simulink model "SC_Eco_5_5"  (R2013a)
settings: Solver=FixedStepDiscrete  StartTime=0.0  StopTime=800  RelTol=1e-3
values from neighbouring files (symbols this model uses):
  T = 1    [Variaveis.mat]
undefined symbols (not defined in the file or in its folder): mu, St
settings Model: Creator=Élio  LastModifiedBy=Élio

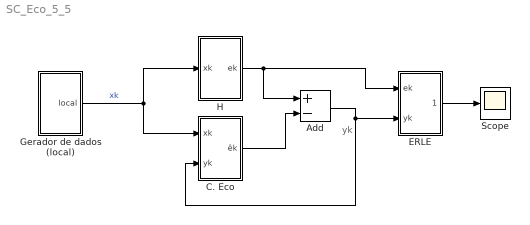
== system SC_Eco_5_5 ==
  note: yk
  Add : Sum  Inputs=+-
  C. Eco : Subsystem
  ERLE : Subsystem
  Gerador de dados (local) : Subsystem
  H : Subsystem
  "Scope " : Scope
  wires:
  Gerador de dados (local)/1(local) -> C. Eco/1(xk), H/1(xk)  "xk"
  C. Eco/1(êk) -> Add/2
  ERLE/1(ERLE) -> "Scope "/1
  H/1(ek) -> ERLE/1(ek), Add/1
  Add/1 -> ERLE/2(yk), C. Eco/2(yk)

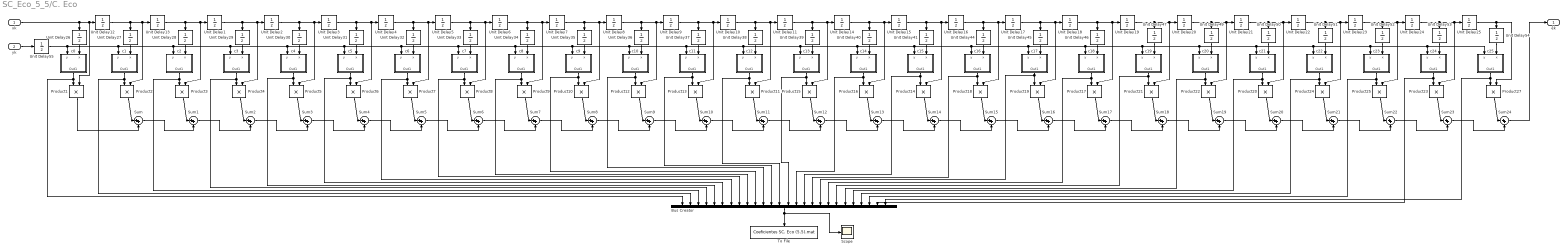
== system SC_Eco_5_5/C. Eco ==
  xk : Inport
  yk : Inport  Port=2
  Bus Creator : BusCreator  Inputs=26
  Product{1..25,27} (26 alike) : Product
  Scope : Scope
  Sum{,1..24} (25 alike) : Sum  Inputs=|++
  To File : ToFile  Filename=Coeficientes SC. Eco (5.5).mat  MatrixName=c5_5  SaveFormat=Timeseries
  Unit Delay{1..41,44..47,49..55} (52 alike) : UnitDelay  SampleTime=-1
  c0 : Subsystem
  c1 : Subsystem
  c10 : Subsystem
  c11 : Subsystem
  c12 : Subsystem
  c13 : Subsystem
  c14 : Subsystem
  c15 : Subsystem
  c16 : Subsystem
  c17 : Subsystem
  c18 : Subsystem
  c19 : Subsystem
  c2 : Subsystem
  c20 : Subsystem
  c21 : Subsystem
  c22 : Subsystem
  c23 : Subsystem
  c24 : Subsystem
  c25 : Subsystem
  c3 : Subsystem
  c4 : Subsystem
  c5 : Subsystem
  c6 : Subsystem
  c7 : Subsystem
  c8 : Subsystem
  c9 : Subsystem
  êk : Outport
  wires:
  Sum/1 -> Sum1/2
  Product1/1 -> Sum/2
  Product2/1 -> Sum/1
  Unit Delay12/1 -> Unit Delay27/1, Product2/2, Unit Delay13/1
  Product3/1 -> Sum1/1
  Product4/1 -> Sum2/1
  Unit Delay13/1 -> Unit Delay1/1, Product3/2, Unit Delay28/1
  Sum2/1 -> Sum3/2
  Product6/1 -> Sum4/1
  xk/1 -> Product1/2, Unit Delay12/1, Unit Delay26/1
  Product5/1 -> Sum3/1
  Sum3/1 -> Sum4/2
  Sum4/1 -> Sum5/2
  Product7/1 -> Sum5/1
  Unit Delay4/1 -> Unit Delay5/1, Product7/2, Unit Delay32/1
  Unit Delay2/1 -> Unit Delay3/1, Product5/2, Unit Delay30/1
  Unit Delay3/1 -> Unit Delay4/1, Product6/2, Unit Delay31/1
  Sum5/1 -> Sum6/2
  Unit Delay5/1 -> Unit Delay6/1, Product8/2, Unit Delay33/1
  Product9/1 -> Sum7/1
  Unit Delay6/1 -> Unit Delay7/1, Product9/2, Unit Delay34/1
  Sum1/1 -> Sum2/2
  Product8/1 -> Sum6/1
  Sum7/1 -> Sum8/2
  Product10/1 -> Sum8/1
  Unit Delay1/1 -> Unit Delay2/1, Product4/2, Unit Delay29/1
  Sum6/1 -> Sum7/2
  Product12/1 -> Sum9/1
  Unit Delay11/1 -> Unit Delay14/1, Product15/2, Unit Delay39/1
  Unit Delay10/1 -> Unit Delay11/1, Product11/2, Unit Delay38/1
  Unit Delay9/1 -> Unit Delay10/1, Product13/2, Unit Delay37/1
  Product11/1 -> Sum11/1
  Product13/1 -> Sum10/1
  Sum12/1 -> Sum13/2
  Product15/1 -> Sum12/1
  Sum9/1 -> Sum10/2
  Product16/1 -> Sum13/1
  Sum11/1 -> Sum12/2
  Sum8/1 -> Sum9/2
  Unit Delay8/1 -> Unit Delay9/1, Product12/2, Unit Delay36/1
  Sum10/1 -> Sum11/2
  Sum13/1 -> Sum14/2
  Unit Delay7/1 -> Unit Delay8/1, Product10/2, Unit Delay35/1
  Unit Delay14/1 -> Unit Delay15/1, Product16/2, Unit Delay40/1
  Product14/1 -> Sum14/1
  Unit Delay17/1 -> Unit Delay18/1, Product19/2, Unit Delay45/1
  Product18/1 -> Sum15/1
  Unit Delay19/1 -> Unit Delay20/1, Product21/2, Unit Delay47/1
  Unit Delay15/1 -> Unit Delay16/1, Product14/2, Unit Delay41/1
  Sum18/1 -> Sum19/2
  Sum16/1 -> Sum17/2
  Product19/1 -> Sum16/1
  Sum21/1 -> Sum22/2
  Sum15/1 -> Sum16/2
  Unit Delay16/1 -> Unit Delay17/1, Product18/2, Unit Delay44/1
  Unit Delay20/1 -> Unit Delay21/1, Product22/2, Unit Delay49/1
  Product21/1 -> Sum18/1
  Sum17/1 -> Sum18/2
  Sum14/1 -> Sum15/2
  Sum19/1 -> Sum20/2
  Product17/1 -> Sum17/1
  Unit Delay22/1 -> Unit Delay23/1, Product24/2, Unit Delay51/1
  Product20/1 -> Sum20/1
  Product24/1 -> Sum21/1
  Unit Delay21/1 -> Unit Delay22/1, Product20/2, Unit Delay50/1
  Sum20/1 -> Sum21/2
  Unit Delay18/1 -> Unit Delay19/1, Product17/2, Unit Delay46/1
  Product22/1 -> Sum19/1
  Unit Delay40/1 -> c14/2(x)
  Unit Delay32/1 -> c6/2(x)
  Product23/1 -> Sum23/1
  Unit Delay24/1 -> Unit Delay25/1, Product23/2, Unit Delay53/1
  Product25/1 -> Sum22/1
  Unit Delay27/1 -> c1/2(x)
  Unit Delay26/1 -> c0/2(x)
  Unit Delay33/1 -> c7/2(x)
  Unit Delay34/1 -> c8/2(x)
  Unit Delay23/1 -> Unit Delay24/1, Product25/2, Unit Delay52/1
  Sum23/1 -> Sum24/2
  Unit Delay28/1 -> c2/2(x)
  Unit Delay35/1 -> c9/2(x)
  Unit Delay36/1 -> c10/2(x)
  Unit Delay44/1 -> c16/2(x)
  Unit Delay45/1 -> c17/2(x)
  Unit Delay46/1 -> c18/2(x)
  Unit Delay25/1 -> Product27/2, Unit Delay54/1
  yk/1 -> Unit Delay55/1
  Sum24/1 -> êk/1
  Unit Delay31/1 -> c5/2(x)
  Unit Delay39/1 -> c13/2(x)
  Unit Delay30/1 -> c4/2(x)
  Unit Delay38/1 -> c12/2(x)
  Unit Delay41/1 -> c15/2(x)
  Unit Delay29/1 -> c3/2(x)
  Unit Delay37/1 -> c11/2(x)
  Sum22/1 -> Sum23/2
  Product27/1 -> Sum24/1
  Unit Delay53/1 -> c24/2(x)
  Unit Delay47/1 -> c19/2(x)
  Unit Delay54/1 -> c25/2(x)
  Unit Delay49/1 -> c20/2(x)
  Unit Delay50/1 -> c21/2(x)
  Unit Delay55/1 -> c0/1(y), c1/1(y), c2/1(y), c3/1(y), c4/1(y), c5/1(y), c6/1(y), c7/1(y), c8/1(y), c9/1(y), c10/1(y), c11/1(y), c12/1(y), c14/1(y), c15/1(y), c16/1(y), c17/1(y), c18/1(y), c19/1(y), c20/1(y), c21/1(y), c22/1(y), c23/1(y), c25/1(y), c24/1(y), c13/1(y)
  Unit Delay52/1 -> c23/2(x)
  Unit Delay51/1 -> c22/2(x)
  c1/1(Out1) -> Bus Creator/2, Product2/1
  c0/1(Out1) -> Bus Creator/1, Product1/1
  c2/1(Out1) -> Bus Creator/3, Product3/1
  c3/1(Out1) -> Bus Creator/4, Product4/1
  c4/1(Out1) -> Bus Creator/5, Product5/1
  c5/1(Out1) -> Bus Creator/6, Product6/1
  c6/1(Out1) -> Bus Creator/7, Product7/1
  c7/1(Out1) -> Bus Creator/8, Product8/1
  c8/1(Out1) -> Bus Creator/9, Product9/1
  c9/1(Out1) -> Bus Creator/10, Product10/1
  c10/1(Out1) -> Bus Creator/11, Product12/1
  c11/1(Out1) -> Bus Creator/12, Product13/1
  c12/1(Out1) -> Bus Creator/13, Product11/1
  c13/1(Out1) -> Bus Creator/14, Product15/1
  c14/1(Out1) -> Bus Creator/15, Product16/1
  c15/1(Out1) -> Bus Creator/16, Product14/1
  c16/1(Out1) -> Bus Creator/17, Product18/1
  c17/1(Out1) -> Bus Creator/18, Product19/1
  c18/1(Out1) -> Bus Creator/19, Product17/1
  c19/1(Out1) -> Bus Creator/20, Product21/1
  c20/1(Out1) -> Bus Creator/21, Product22/1
  c21/1(Out1) -> Bus Creator/22, Product20/1
  c22/1(Out1) -> Bus Creator/23, Product24/1
  c23/1(Out1) -> Bus Creator/24, Product25/1
  c24/1(Out1) -> Bus Creator/25, Product23/1
  c25/1(Out1) -> Bus Creator/26, Product27/1
  Bus Creator/1 -> Scope/1, To File/1

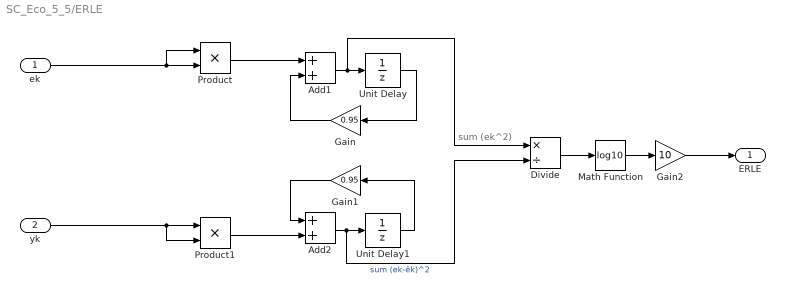
== system SC_Eco_5_5/ERLE ==
  note: sum (ek^2)
  ek : Inport
  yk : Inport  Port=2
  Add1 : Sum  RequirementInfo={} %GIDa_ce1c1d54_3b96_46b2_aaba_1a46e1338465
  Add2 : Sum  RequirementInfo={} %GIDa_00d8fe9e_6752_48b6_b576_e88cd44475ea
  Divide : Product  Inputs=*/
  Gain : Gain  Gain=0.95
  Gain1 : Gain  Gain=0.95
  Gain2 : Gain  Gain=10
  Math Function : Math  Operator=log10  SaturateOnIntegerOverflow=on
  Product : Product
  Product1 : Product
  Unit Delay : UnitDelay  SampleTime=-1
  Unit Delay1 : UnitDelay  SampleTime=-1
  ERLE : Outport
  wires:
  yk/1 -> Product1/2, Product1/1
  Math Function/1 -> Gain2/1
  Add2/1 -> Divide/2, Unit Delay1/1  "sum (ek-êk)^2"
  Product/1 -> Add1/1
  Gain1/1 -> Add2/1
  Divide/1 -> Math Function/1
  Gain2/1 -> ERLE/1
  Unit Delay1/1 -> Gain1/1
  Add1/1 -> Divide/1, Unit Delay/1
  Unit Delay/1 -> Gain/1
  ek/1 -> Product/2, Product/1
  Gain/1 -> Add1/2
  Product1/1 -> Add2/2

== system SC_Eco_5_5/Gerador de dados (local) ==
  Conversor de nível : Subsystem
  Pulse Generator : DiscretePulseGenerator  PulseType=Time based  Period=2*T  PulseWidth=50  SampleTime=St
  Scrambler (local) : Subsystem
  local : Outport
  wires:
  Pulse Generator/1 -> Scrambler (local)/1(In1)
  Conversor de nível/1(Out2) -> local/1
  Scrambler (local)/1(Out1) -> Conversor de nível/1(In2)

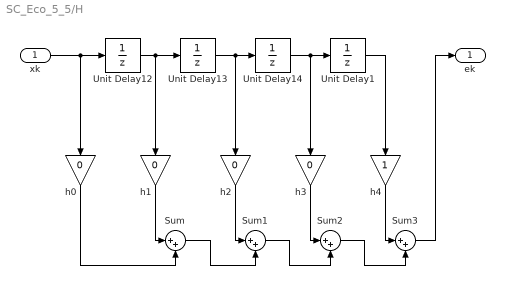
== system SC_Eco_5_5/H ==
  xk : Inport
  Sum{,1..3} (4 alike) : Sum  Inputs=|++
  Unit Delay{1,12..14} (4 alike) : UnitDelay  SampleTime=-1
  h{0..3} (4 alike) : Gain  Gain=0
  h4 : Gain
  ek : Outport
  wires:
  Sum3/1 -> ek/1
  xk/1 -> Unit Delay12/1, h0/1
  Unit Delay13/1 -> Unit Delay14/1, h2/1
  h3/1 -> Sum2/1
  Unit Delay14/1 -> Unit Delay1/1, h3/1
  Sum/1 -> Sum1/2
  h2/1 -> Sum1/1
  h0/1 -> Sum/2
  Unit Delay12/1 -> Unit Delay13/1, h1/1
  Sum1/1 -> Sum2/2
  h1/1 -> Sum/1
  Unit Delay1/1 -> h4/1
  Sum2/1 -> Sum3/2
  h4/1 -> Sum3/1

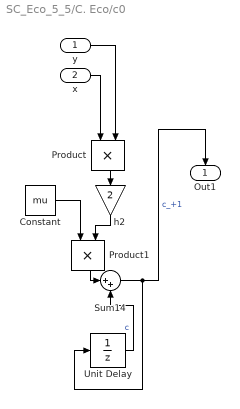
== system SC_Eco_5_5/C. Eco/c0 ==
  y : Inport
  x : Inport  Port=2
  Constant : Constant  Value=mu
  Product : Product
  Product1 : Product
  Sum14 : Sum  Inputs=|++
  "Unit Delay " : UnitDelay  SampleTime=-1
  h2 : Gain  Gain=2
  Out1 : Outport
  wires:
  x/1 -> Product/1
  Sum14/1 -> Out1/1, "Unit Delay "/1  "c_+1"
  "Unit Delay "/1 -> Sum14/2  "c"
  Product/1 -> h2/1
  y/1 -> Product/2
  Product1/1 -> Sum14/1
  h2/1 -> Product1/2
  Constant/1 -> Product1/1

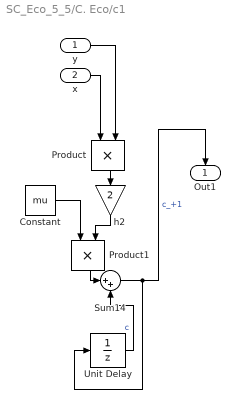
== system SC_Eco_5_5/C. Eco/c1 ==
  y : Inport
  x : Inport  Port=2
  Constant : Constant  Value=mu
  Product : Product
  Product1 : Product
  Sum14 : Sum  Inputs=|++
  "Unit Delay " : UnitDelay  SampleTime=-1
  h2 : Gain  Gain=2
  Out1 : Outport
  wires:
  x/1 -> Product/1
  Sum14/1 -> Out1/1, "Unit Delay "/1  "c_+1"
  "Unit Delay "/1 -> Sum14/2  "c"
  Product/1 -> h2/1
  y/1 -> Product/2
  Product1/1 -> Sum14/1
  h2/1 -> Product1/2
  Constant/1 -> Product1/1

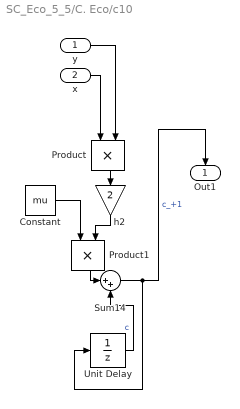
== system SC_Eco_5_5/C. Eco/c10 ==
  y : Inport
  x : Inport  Port=2
  Constant : Constant  Value=mu
  Product : Product
  Product1 : Product
  Sum14 : Sum  Inputs=|++
  "Unit Delay " : UnitDelay  SampleTime=-1
  h2 : Gain  Gain=2
  Out1 : Outport
  wires:
  x/1 -> Product/1
  Sum14/1 -> Out1/1, "Unit Delay "/1  "c_+1"
  "Unit Delay "/1 -> Sum14/2  "c"
  Product/1 -> h2/1
  y/1 -> Product/2
  Product1/1 -> Sum14/1
  h2/1 -> Product1/2
  Constant/1 -> Product1/1

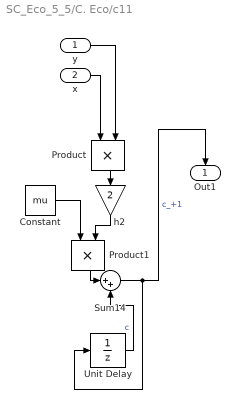
== system SC_Eco_5_5/C. Eco/c11 ==
  y : Inport
  x : Inport  Port=2
  Constant : Constant  Value=mu
  Product : Product
  Product1 : Product
  Sum14 : Sum  Inputs=|++
  "Unit Delay " : UnitDelay  SampleTime=-1
  h2 : Gain  Gain=2
  Out1 : Outport
  wires:
  x/1 -> Product/1
  Sum14/1 -> Out1/1, "Unit Delay "/1  "c_+1"
  "Unit Delay "/1 -> Sum14/2  "c"
  Product/1 -> h2/1
  y/1 -> Product/2
  Product1/1 -> Sum14/1
  h2/1 -> Product1/2
  Constant/1 -> Product1/1

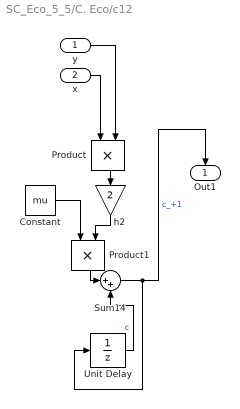
== system SC_Eco_5_5/C. Eco/c12 ==
  y : Inport
  x : Inport  Port=2
  Constant : Constant  Value=mu
  Product : Product
  Product1 : Product
  Sum14 : Sum  Inputs=|++
  "Unit Delay " : UnitDelay  SampleTime=-1
  h2 : Gain  Gain=2
  Out1 : Outport
  wires:
  x/1 -> Product/1
  Sum14/1 -> Out1/1, "Unit Delay "/1  "c_+1"
  "Unit Delay "/1 -> Sum14/2  "c"
  Product/1 -> h2/1
  y/1 -> Product/2
  Product1/1 -> Sum14/1
  h2/1 -> Product1/2
  Constant/1 -> Product1/1

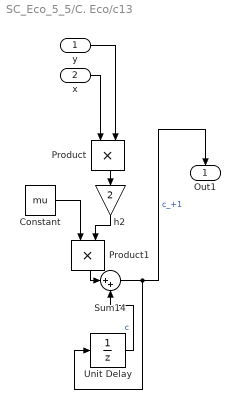
== system SC_Eco_5_5/C. Eco/c13 ==
  y : Inport
  x : Inport  Port=2
  Constant : Constant  Value=mu
  Product : Product
  Product1 : Product
  Sum14 : Sum  Inputs=|++
  "Unit Delay " : UnitDelay  SampleTime=-1
  h2 : Gain  Gain=2
  Out1 : Outport
  wires:
  x/1 -> Product/1
  Sum14/1 -> Out1/1, "Unit Delay "/1  "c_+1"
  "Unit Delay "/1 -> Sum14/2  "c"
  Product/1 -> h2/1
  y/1 -> Product/2
  Product1/1 -> Sum14/1
  h2/1 -> Product1/2
  Constant/1 -> Product1/1

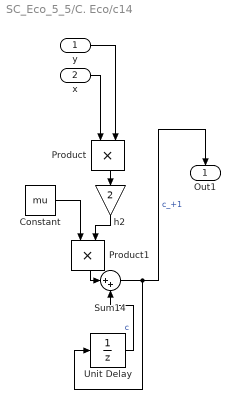
== system SC_Eco_5_5/C. Eco/c14 ==
  y : Inport
  x : Inport  Port=2
  Constant : Constant  Value=mu
  Product : Product
  Product1 : Product
  Sum14 : Sum  Inputs=|++
  "Unit Delay " : UnitDelay  SampleTime=-1
  h2 : Gain  Gain=2
  Out1 : Outport
  wires:
  x/1 -> Product/1
  Sum14/1 -> Out1/1, "Unit Delay "/1  "c_+1"
  "Unit Delay "/1 -> Sum14/2  "c"
  Product/1 -> h2/1
  y/1 -> Product/2
  Product1/1 -> Sum14/1
  h2/1 -> Product1/2
  Constant/1 -> Product1/1

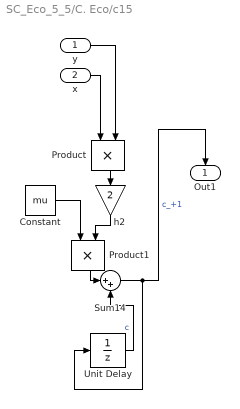
== system SC_Eco_5_5/C. Eco/c15 ==
  y : Inport
  x : Inport  Port=2
  Constant : Constant  Value=mu
  Product : Product
  Product1 : Product
  Sum14 : Sum  Inputs=|++
  "Unit Delay " : UnitDelay  SampleTime=-1
  h2 : Gain  Gain=2
  Out1 : Outport
  wires:
  x/1 -> Product/1
  Sum14/1 -> Out1/1, "Unit Delay "/1  "c_+1"
  "Unit Delay "/1 -> Sum14/2  "c"
  Product/1 -> h2/1
  y/1 -> Product/2
  Product1/1 -> Sum14/1
  h2/1 -> Product1/2
  Constant/1 -> Product1/1

== system SC_Eco_5_5/C. Eco/c16 ==
  y : Inport
  x : Inport  Port=2
  Constant : Constant  Value=mu
  Product : Product
  Product1 : Product
  Sum14 : Sum  Inputs=|++
  "Unit Delay " : UnitDelay  SampleTime=-1
  h2 : Gain  Gain=2
  Out1 : Outport
  wires:
  x/1 -> Product/1
  Sum14/1 -> Out1/1, "Unit Delay "/1  "c_+1"
  "Unit Delay "/1 -> Sum14/2  "c"
  Product/1 -> h2/1
  y/1 -> Product/2
  Product1/1 -> Sum14/1
  h2/1 -> Product1/2
  Constant/1 -> Product1/1

== system SC_Eco_5_5/C. Eco/c17 ==
  y : Inport
  x : Inport  Port=2
  Constant : Constant  Value=mu
  Product : Product
  Product1 : Product
  Sum14 : Sum  Inputs=|++
  "Unit Delay " : UnitDelay  SampleTime=-1
  h2 : Gain  Gain=2
  Out1 : Outport
  wires:
  x/1 -> Product/1
  Sum14/1 -> Out1/1, "Unit Delay "/1  "c_+1"
  "Unit Delay "/1 -> Sum14/2  "c"
  Product/1 -> h2/1
  y/1 -> Product/2
  Product1/1 -> Sum14/1
  h2/1 -> Product1/2
  Constant/1 -> Product1/1

== system SC_Eco_5_5/C. Eco/c18 ==
  y : Inport
  x : Inport  Port=2
  Constant : Constant  Value=mu
  Product : Product
  Product1 : Product
  Sum14 : Sum  Inputs=|++
  "Unit Delay " : UnitDelay  SampleTime=-1
  h2 : Gain  Gain=2
  Out1 : Outport
  wires:
  x/1 -> Product/1
  Sum14/1 -> Out1/1, "Unit Delay "/1  "c_+1"
  "Unit Delay "/1 -> Sum14/2  "c"
  Product/1 -> h2/1
  y/1 -> Product/2
  Product1/1 -> Sum14/1
  h2/1 -> Product1/2
  Constant/1 -> Product1/1

== system SC_Eco_5_5/C. Eco/c19 ==
  y : Inport
  x : Inport  Port=2
  Constant : Constant  Value=mu
  Product : Product
  Product1 : Product
  Sum14 : Sum  Inputs=|++
  "Unit Delay " : UnitDelay  SampleTime=-1
  h2 : Gain  Gain=2
  Out1 : Outport
  wires:
  x/1 -> Product/1
  Sum14/1 -> Out1/1, "Unit Delay "/1  "c_+1"
  "Unit Delay "/1 -> Sum14/2  "c"
  Product/1 -> h2/1
  y/1 -> Product/2
  Product1/1 -> Sum14/1
  h2/1 -> Product1/2
  Constant/1 -> Product1/1

== system SC_Eco_5_5/C. Eco/c2 ==
  y : Inport
  x : Inport  Port=2
  Constant : Constant  Value=mu
  Product : Product
  Product1 : Product
  Sum14 : Sum  Inputs=|++
  "Unit Delay " : UnitDelay  SampleTime=-1
  h2 : Gain  Gain=2
  Out1 : Outport
  wires:
  x/1 -> Product/1
  Sum14/1 -> Out1/1, "Unit Delay "/1  "c_+1"
  "Unit Delay "/1 -> Sum14/2  "c"
  Product/1 -> h2/1
  y/1 -> Product/2
  Product1/1 -> Sum14/1
  h2/1 -> Product1/2
  Constant/1 -> Product1/1

== system SC_Eco_5_5/C. Eco/c20 ==
  y : Inport
  x : Inport  Port=2
  Constant : Constant  Value=mu
  Product : Product
  Product1 : Product
  Sum14 : Sum  Inputs=|++
  "Unit Delay " : UnitDelay  SampleTime=-1
  h2 : Gain  Gain=2
  Out1 : Outport
  wires:
  x/1 -> Product/1
  Sum14/1 -> Out1/1, "Unit Delay "/1  "c_+1"
  "Unit Delay "/1 -> Sum14/2  "c"
  Product/1 -> h2/1
  y/1 -> Product/2
  Product1/1 -> Sum14/1
  h2/1 -> Product1/2
  Constant/1 -> Product1/1

== system SC_Eco_5_5/C. Eco/c21 ==
  y : Inport
  x : Inport  Port=2
  Constant : Constant  Value=mu
  Product : Product
  Product1 : Product
  Sum14 : Sum  Inputs=|++
  "Unit Delay " : UnitDelay  SampleTime=-1
  h2 : Gain  Gain=2
  Out1 : Outport
  wires:
  x/1 -> Product/1
  Sum14/1 -> Out1/1, "Unit Delay "/1  "c_+1"
  "Unit Delay "/1 -> Sum14/2  "c"
  Product/1 -> h2/1
  y/1 -> Product/2
  Product1/1 -> Sum14/1
  h2/1 -> Product1/2
  Constant/1 -> Product1/1

== system SC_Eco_5_5/C. Eco/c22 ==
  y : Inport
  x : Inport  Port=2
  Constant : Constant  Value=mu
  Product : Product
  Product1 : Product
  Sum14 : Sum  Inputs=|++
  "Unit Delay " : UnitDelay  SampleTime=-1
  h2 : Gain  Gain=2
  Out1 : Outport
  wires:
  x/1 -> Product/1
  Sum14/1 -> Out1/1, "Unit Delay "/1  "c_+1"
  "Unit Delay "/1 -> Sum14/2  "c"
  Product/1 -> h2/1
  y/1 -> Product/2
  Product1/1 -> Sum14/1
  h2/1 -> Product1/2
  Constant/1 -> Product1/1

== system SC_Eco_5_5/C. Eco/c23 ==
  y : Inport
  x : Inport  Port=2
  Constant : Constant  Value=mu
  Product : Product
  Product1 : Product
  Sum14 : Sum  Inputs=|++
  "Unit Delay " : UnitDelay  SampleTime=-1
  h2 : Gain  Gain=2
  Out1 : Outport
  wires:
  x/1 -> Product/1
  Sum14/1 -> Out1/1, "Unit Delay "/1  "c_+1"
  "Unit Delay "/1 -> Sum14/2  "c"
  Product/1 -> h2/1
  y/1 -> Product/2
  Product1/1 -> Sum14/1
  h2/1 -> Product1/2
  Constant/1 -> Product1/1

== system SC_Eco_5_5/C. Eco/c24 ==
  y : Inport
  x : Inport  Port=2
  Constant : Constant  Value=mu
  Product : Product
  Product1 : Product
  Sum14 : Sum  Inputs=|++
  "Unit Delay " : UnitDelay  SampleTime=-1
  h2 : Gain  Gain=2
  Out1 : Outport
  wires:
  x/1 -> Product/1
  Sum14/1 -> Out1/1, "Unit Delay "/1  "c_+1"
  "Unit Delay "/1 -> Sum14/2  "c"
  Product/1 -> h2/1
  y/1 -> Product/2
  Product1/1 -> Sum14/1
  h2/1 -> Product1/2
  Constant/1 -> Product1/1

== system SC_Eco_5_5/C. Eco/c25 ==
  y : Inport
  x : Inport  Port=2
  Constant : Constant  Value=mu
  Product : Product
  Product1 : Product
  Sum14 : Sum  Inputs=|++
  "Unit Delay " : UnitDelay  SampleTime=-1
  h2 : Gain  Gain=2
  Out1 : Outport
  wires:
  x/1 -> Product/1
  Sum14/1 -> Out1/1, "Unit Delay "/1  "c_+1"
  "Unit Delay "/1 -> Sum14/2  "c"
  Product/1 -> h2/1
  y/1 -> Product/2
  Product1/1 -> Sum14/1
  h2/1 -> Product1/2
  Constant/1 -> Product1/1

== system SC_Eco_5_5/C. Eco/c3 ==
  y : Inport
  x : Inport  Port=2
  Constant : Constant  Value=mu
  Product : Product
  Product1 : Product
  Sum14 : Sum  Inputs=|++
  "Unit Delay " : UnitDelay  SampleTime=-1
  h2 : Gain  Gain=2
  Out1 : Outport
  wires:
  x/1 -> Product/1
  Sum14/1 -> Out1/1, "Unit Delay "/1  "c_+1"
  "Unit Delay "/1 -> Sum14/2  "c"
  Product/1 -> h2/1
  y/1 -> Product/2
  Product1/1 -> Sum14/1
  h2/1 -> Product1/2
  Constant/1 -> Product1/1

== system SC_Eco_5_5/C. Eco/c4 ==
  y : Inport
  x : Inport  Port=2
  Constant : Constant  Value=mu
  Product : Product
  Product1 : Product
  Sum14 : Sum  Inputs=|++
  "Unit Delay " : UnitDelay  SampleTime=-1
  h2 : Gain  Gain=2
  Out1 : Outport
  wires:
  x/1 -> Product/1
  Sum14/1 -> Out1/1, "Unit Delay "/1  "c_+1"
  "Unit Delay "/1 -> Sum14/2  "c"
  Product/1 -> h2/1
  y/1 -> Product/2
  Product1/1 -> Sum14/1
  h2/1 -> Product1/2
  Constant/1 -> Product1/1

== system SC_Eco_5_5/C. Eco/c5 ==
  y : Inport
  x : Inport  Port=2
  Constant : Constant  Value=mu
  Product : Product
  Product1 : Product
  Sum14 : Sum  Inputs=|++
  "Unit Delay " : UnitDelay  SampleTime=-1
  h2 : Gain  Gain=2
  Out1 : Outport
  wires:
  x/1 -> Product/1
  Sum14/1 -> Out1/1, "Unit Delay "/1  "c_+1"
  "Unit Delay "/1 -> Sum14/2  "c"
  Product/1 -> h2/1
  y/1 -> Product/2
  Product1/1 -> Sum14/1
  h2/1 -> Product1/2
  Constant/1 -> Product1/1

== system SC_Eco_5_5/C. Eco/c6 ==
  y : Inport
  x : Inport  Port=2
  Constant : Constant  Value=mu
  Product : Product
  Product1 : Product
  Sum14 : Sum  Inputs=|++
  "Unit Delay " : UnitDelay  SampleTime=-1
  h2 : Gain  Gain=2
  Out1 : Outport
  wires:
  x/1 -> Product/1
  Sum14/1 -> Out1/1, "Unit Delay "/1  "c_+1"
  "Unit Delay "/1 -> Sum14/2  "c"
  Product/1 -> h2/1
  y/1 -> Product/2
  Product1/1 -> Sum14/1
  h2/1 -> Product1/2
  Constant/1 -> Product1/1

== system SC_Eco_5_5/C. Eco/c7 ==
  y : Inport
  x : Inport  Port=2
  Constant : Constant  Value=mu
  Product : Product
  Product1 : Product
  Sum14 : Sum  Inputs=|++
  "Unit Delay " : UnitDelay  SampleTime=-1
  h2 : Gain  Gain=2
  Out1 : Outport
  wires:
  x/1 -> Product/1
  Sum14/1 -> Out1/1, "Unit Delay "/1  "c_+1"
  "Unit Delay "/1 -> Sum14/2  "c"
  Product/1 -> h2/1
  y/1 -> Product/2
  Product1/1 -> Sum14/1
  h2/1 -> Product1/2
  Constant/1 -> Product1/1

== system SC_Eco_5_5/C. Eco/c8 ==
  y : Inport
  x : Inport  Port=2
  Constant : Constant  Value=mu
  Product : Product
  Product1 : Product
  Sum14 : Sum  Inputs=|++
  "Unit Delay " : UnitDelay  SampleTime=-1
  h2 : Gain  Gain=2
  Out1 : Outport
  wires:
  x/1 -> Product/1
  Sum14/1 -> Out1/1, "Unit Delay "/1  "c_+1"
  "Unit Delay "/1 -> Sum14/2  "c"
  Product/1 -> h2/1
  y/1 -> Product/2
  Product1/1 -> Sum14/1
  h2/1 -> Product1/2
  Constant/1 -> Product1/1

== system SC_Eco_5_5/C. Eco/c9 ==
  y : Inport
  x : Inport  Port=2
  Constant : Constant  Value=mu
  Product : Product
  Product1 : Product
  Sum14 : Sum  Inputs=|++
  "Unit Delay " : UnitDelay  SampleTime=-1
  h2 : Gain  Gain=2
  Out1 : Outport
  wires:
  x/1 -> Product/1
  Sum14/1 -> Out1/1, "Unit Delay "/1  "c_+1"
  "Unit Delay "/1 -> Sum14/2  "c"
  Product/1 -> h2/1
  y/1 -> Product/2
  Product1/1 -> Sum14/1
  h2/1 -> Product1/2
  Constant/1 -> Product1/1

== system SC_Eco_5_5/Gerador de dados (local)/Conversor de nível ==
  In2 : Inport
  Constant : Constant  Value=-1
  Gain1 : Gain  Gain=2
  Sum : Sum  Inputs=++|
  Out2 : Outport
  wires:
  In2/1 -> Gain1/1
  Sum/1 -> Out2/1
  Gain1/1 -> Sum/2
  Constant/1 -> Sum/1

== system SC_Eco_5_5/Gerador de dados (local)/Scrambler (local) ==
  In1 : Inport
  Logical Operator : Logic  Operator=XOR  AllPortsSameDT=off  OutDataTypeStr=fixdt(1,16)
  Logical Operator1 : Logic  Operator=XOR  AllPortsSameDT=off  OutDataTypeStr=boolean
  Unit Delay{,1..4} (5 alike) : UnitDelay  SampleTime=-1
  Out1 : Outport
  wires:
  In1/1 -> Logical Operator/1
  Logical Operator/1 -> Out1/1, Unit Delay/1
  Unit Delay/1 -> Unit Delay1/1
  Logical Operator1/1 -> Logical Operator/2
  Unit Delay3/1 -> Unit Delay4/1
  Unit Delay4/1 -> Logical Operator1/2
  Unit Delay1/1 -> Unit Delay2/1
  Unit Delay2/1 -> Logical Operator1/1, Unit Delay3/1
